simulink model "ecg_modelo_i"  (Simulink 8.1)
settings: Solver=ode4  StartTime=0.0  StopTime=10  FixedStep=Ts  RelTol=1e-3
undefined symbols (not defined in the file): dfilt, Ts
libraries: dsparch4 x1, commnoisgen2 x1
Description:
  | Real-Time Signal Generator
  | 
  | This demonstration shows how to produce an analog output signal using
  | Real-Time Windows Target. Because analog output typically requires
  | less configuration and is easier to connect than analog input, this demo
  | is a good start to your experiments with data acquisition boards. You can
  | verify the presence of the generated signal e.g. by connecting an
  | oscilloscope to the analog output pins of your data acquisition board.
  | 
  | How to run this demo:
  | 
  |   1. Open the Analog Output block and select your data acquisition board.
  |       If there's no board installed, install it using the Install new board button.
  |   2. Build the model using Tools -> Code Generation -> Build Model.
  |   3. Connect to the real-time code using Simulation -> Connect to target.
  |   4. Start the real-time execution using Simulation -> Start real-time code.
  | 
  | Note:
  | To run this demo, you must have a data acquisition board plugged into your computer.
settings Model: Creator=The MathWorks Inc.  LastModifiedBy=rafa  ExtModeTrigType=signal  ExtModeTrigLevel=0.500000
settings DataIOCC: SignalLoggingName=logsOut
settings OptimizationCC: InitFltsAndDblsToZero=on  EfficientMapNaN2IntZero=off
settings DebuggingCC: SignalResolutionControl=TryResolveAllWithWarning  SolverPrmCheckMsg=none  StrictBusMsg=Warning
settings HardwareCC: ProdIntDivRoundTo=Zero  ProdEndianess=LittleEndian  ProdHWDeviceType=32-bit Real-Time Windows Target
settings RTWCC: SystemTargetFile=rtwin.tlc  TemplateMakefile=rtwin.tmf  Description=Real-Time Windows Target  ProcessScript=rtwin_make_rtw_hook
settings TargetCC: TargetLibSuffix=_rtwin.lib  TargetPreCompLibLocation=C:\Program Files\MATLAB\R2011a\toolbox\rtw\targets\rtwin\lib\win32  CodeReplacementLibrary=ANSI_C  IsPILTarget=off  EnableShiftOperators=on
settings CustomProperty: DataType=string

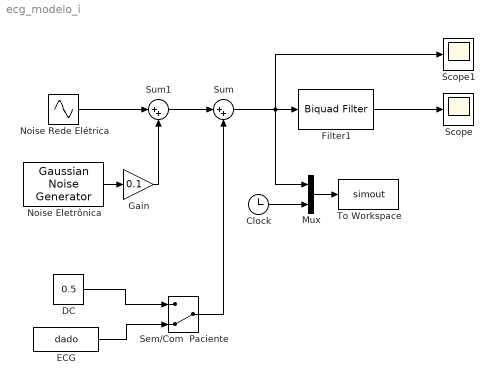
== system ecg_modelo_i ==
  Clock : Clock
  DC : Constant  Value=0.5
  ECG : FromWorkspace  VariableName=dado  SampleTime=Ts  Interpolate=off  OutputAfterFinalValue=Cyclic repetition
  Filter1 : dsparch4/Biquad Filter  Tag=BlockMethodSubSystem  IIRFiltStruct=Direct form II  CoeffSource=Specify via dialog  BiQuadCoeffs=[1 2 1 1 -1.86462554633674582 0.925106300799211634;1 2 1 1 -1.74064279640538611 0.797102062333109984;1 2 1 1 -1.64745998107697678 0.700896781188402596;1 2 1 1 -1.5857819253944847 0.637218144022521638;1 2 1 1 -1.5551723015747918 0.605615670380480253]  a0Flag=Warning  IC=0  ICnum=0  ICden=0  denAccumFracLength=30  denProdOutputFracLength=30  secondMemoryFracLength=15  roundingMode=Floor  overflowMode=off  ScaleValues=[0.0151201886156164568;0.0141148164819310078;0.0133592000278565052;0.0128590546570092942;0.0126108422014221191;1]  optimizeScaleValues=on  ScaleValueMode=Specify via input port (g)  scaleValueFracLength=14  FilterSource=Specify via dialog  dfiltObjectName=dfilt.df2tsos([1 0.3 0.4],[1 0.1 0.2])
  Gain : Gain  Gain=0.1
  Mux : Mux  Inputs=2
  Noise Eletrônica : commnoisgen2/Gaussian Noise Generator  m=0  d=1  s=41  Ts=Ts  frameBased=off  sampPerFrame=1  orient=off  outDataType=double
  Noise Rede Elétrica : Sin  Frequency=60*2*pi  Samples=60  SampleTime=Ts
  Scope : Scope
      settings: TimeRange=1000  YMin=-0.11  YMax=0.11
  Scope1 : Scope
      settings: TimeRange=1000  YMin=-0.11  YMax=0.11
  Sem/Com  Paciente : ManualSwitch  CurrentSetting=0
  Sum : Sum  Inputs=|++  SampleTime=Ts
  Sum1 : Sum  Inputs=|++  SampleTime=Ts
  To Workspace : ToWorkspace  VariableName=simout  SampleTime=Ts
  wires:
  Sum/1 -> Filter1/1, Mux/1, Scope1/1
  Mux/1 -> To Workspace/1
  Noise Rede Elétrica/1 -> Sum1/1
  Sum1/1 -> Sum/1
  Noise Eletrônica/1 -> Gain/1
  Gain/1 -> Sum1/2
  Clock/1 -> Mux/2
  ECG/1 -> Sem/Com  Paciente/2
  DC/1 -> Sem/Com  Paciente/1
  Sem/Com  Paciente/1 -> Sum/2
  Filter1/1 -> Scope/1
